simulink model "FBL_UAV_Final_All"  (R2024b)
settings: Solver=ode45  StartTime=0.0  StopTime=3  MaxStep=0.001  RelTol=1e-3
undefined symbols (not defined in the file): A, A_inv, B, Q, R
libraries: slpidlib x8, mpclib x1, rllib x1, simulink x1
(part 2 of 2)

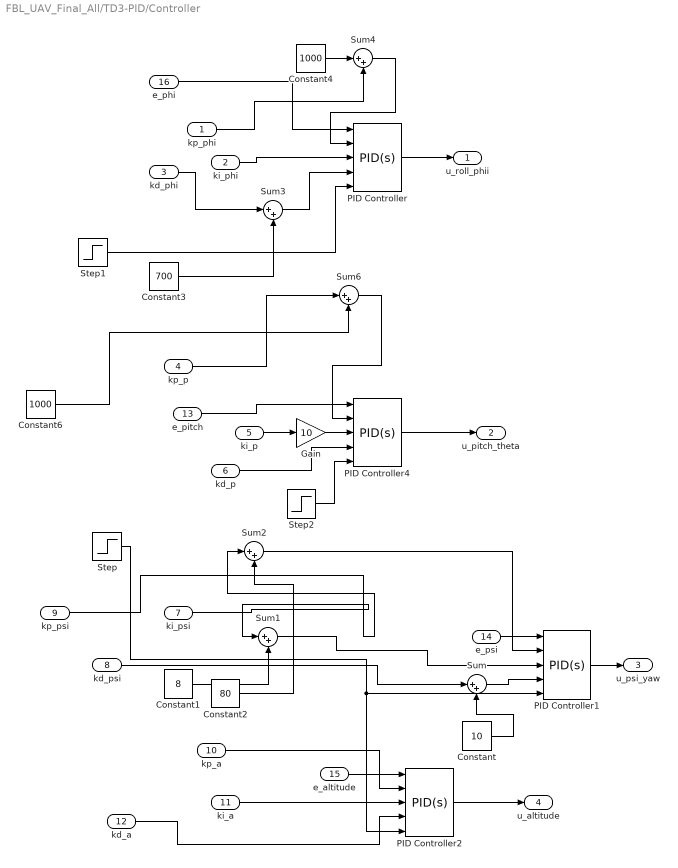
== system FBL_UAV_Final_All/TD3-PID/Controller ==
  kp_phi : Inport
  ki_phi : Inport  Port=2
  kd_phi : Inport  Port=3
  kp_p : Inport  Port=4
  ki_p : Inport  Port=5
  kd_p : Inport  Port=6
  ki_psi : Inport  Port=7
  kd_psi : Inport  Port=8
  kp_psi : Inport  Port=9
  kp_a : Inport  Port=10
  ki_a : Inport  Port=11
  kd_a : Inport  Port=12
  e_pitch : Inport  Port=13
  e_psi : Inport  Port=14
  e_altitude : Inport  Port=15
  e_phi : Inport  Port=16
  Constant : Constant  Value=10
  Constant1 : Constant  Value=8
  Constant2 : Constant  Value=80
  Constant3 : Constant  Value=700
  Constant4 : Constant  Value=1000
  Constant6 : Constant  Value=1000
  Gain : Gain  Gain=10
  PID Controller{,1..2,4} (4 alike) : slpidlib/PID Controller  Controller=PID  Form=Parallel  TimeDomain=Continuous-time  UseExternalTs=off  SampleTime=0.1  IntegratorMethod=Forward Euler  FilterMethod=Forward Euler  ControllerParametersSource=external  P=1  I=1  UseKiTs=off  D=0  UseExternalDerivativeSource=off  N=100  UseFilter=on  TunerSelectOption=Transfer Function Based (PID Tuner App)  InitialConditionSource=internal  InitialConditionForIntegrator=0  InitialConditionForFilter=0  DifferentiatorICPrevScaledInput=0  ExternalReset=none  TrackingMode=off  Kt=1  LimitOutput=off  SatLimitsSource=internal  UpperSaturationLimit=inf  LowerSaturationLimit=-inf  LinearizeAsGain=on  AntiWindupMode=none  Kb=1  LimitIntegrator=off  UpperIntegratorSaturationLimit=inf  LowerIntegratorSaturationLimit=-inf  POutMin=[]  POutMax=[]  IOutMin=[]  IOutMax=[]  DOutMin=[]  DOutMax=[]  NOutMin=[]  NOutMax=[]  SumOutMin=[]  SumOutMax=[]  SaturationOutMin=[]  SaturationOutMax=[]  PParamMin=[]  PParamMax=[]  IParamMin=[]  IParamMax=[]  DParamMin=[]  DParamMax=[]  NParamMin=[]  NParamMax=[]  KbParamMin=[]  KbParamMax=[]  KtParamMin=[]  KtParamMax=[]  KbOutMin=[]  KbOutMax=[]  KtOutMin=[]  KtOutMax=[]  IntegratorOutMin=[]  IntegratorOutMax=[]  FilterOutMin=[]  FilterOutMax=[]  SumI1OutMin=[]  SumI1OutMax=[]  SumI2OutMin=[]  SumI2OutMax=[]  SumI3OutMin=[]  SumI3OutMax=[]  SumI4OutMin=[]  SumI4OutMax=[]  SumDOutMin=[]  SumDOutMax=[]  DifferentiatorOutMin=[]  DifferentiatorOutMax=[]  FilterDiffOutCoefMin=[]  FilterDiffOutCoefMax=[]  ReciprocalOutMin=[]  ReciprocalOutMax=[]  SumDenOutMin=[]  SumDenOutMax=[]  SumNumOutMin=[]  SumNumOutMax=[]  DivideOutMin=[]  DivideOutMax=[]  UdiffTsProdOutMin=[]  UdiffTsProdOutMax=[]  NTsProdOutMin=[]  NTsProdOutMax=[]  UintegralTsProdOutMin=[]  UintegralTsProdOutMax=[]  UngainTsProdOutMin=[]  UngainTsProdOutMax=[]  ClampingZeroOutDataTypeStr=Inherit: Inherit via back propagation  ClampingZeroOutMin=[]  ClampingZeroOutMax=[]  FilterDenConstantOutDataTypeStr=Inherit: Inherit via back propagation  FilterDenConstantOutMin=[]  FilterDenConstantOutMax=[]  PCopyOutDataTypeStr=Inherit: Inherit via back propagation  PCopyOutMin=[]  PCopyOutMax=[]  NCopyOutDataTypeStr=Inherit: Inherit via back propagation  NCopyOutMin=[]  NCopyOutMax=[]  IntegratorContinuousStateAttributes=''  IntegratorStateMustResolveToSignalObject=off  IntegratorRTWStateStorageClass=Auto  FilterContinuousStateAttributes=''  FilterStateMustResolveToSignalObject=off  FilterRTWStateStorageClass=Auto  ParallelPVariant=ExternalParameters  IdealPVariant=Disabled  IVariant=ExternalParameters  DVariant=ExternalParameters  IntegratorVariant=Continuous  SatVariant=Disabled  AWVariant=Passthrough  PCopyVariant=Disabled  TRVariant=Disabled  FdbkBlocksVariant=Forward  IdealPFdbkVariant=Disabled  SatFdbkVariant=Disabled  DerivativeFilterVariant=ContFilter  NVariant=ExternalParameters  NCopyVariant=Disabled  FilterICVariant=InternalICsFilter  IntegratorICVariant=InternalICs  ExternalResetVariant=Disabled  TRSumVariant=Passthrough  SumFdbkVariant=Disabled  SumVariant=Sum_PID  TsampFilterVariant=InternalTs  TsampNgainVariant=Passthrough  TsampIntegralVariant=Disabled_SignalSpec  ExternalSaturationOutDataTypeStr=Inherit: Same as second input  DerivativeSourceVariant=ErrorSignal  PreIntVariant=InternalPreInt
  Step : Step  Time=0  After=800  SampleTime=0.1
  Step1 : Step  Time=0  After=800  SampleTime=0.1
  Step2 : Step  Time=0  After=700  SampleTime=0.1
  Sum{,1..4,6} (6 alike) : Sum  Inputs=|++
  u_roll_phii : Outport
  u_pitch_theta : Outport  Port=2
  u_psi_yaw : Outport  Port=3
  u_altitude : Outport  Port=4
  wires:
  Step/1 -> PID Controller2/5, PID Controller1/5
  e_phi/1 -> PID Controller/1
  PID Controller/1 -> u_roll_phii/1
  PID Controller4/1 -> u_pitch_theta/1
  PID Controller2/1 -> u_altitude/1
  e_altitude/1 -> PID Controller2/1
  e_psi/1 -> PID Controller1/1
  PID Controller1/1 -> u_psi_yaw/1
  kp_a/1 -> PID Controller2/2
  ki_a/1 -> PID Controller2/3
  kd_a/1 -> PID Controller2/4
  kp_psi/1 -> Sum2/1
  ki_psi/1 -> Sum1/1
  kd_psi/1 -> Sum/1
  Constant/1 -> Sum/2
  Sum/1 -> PID Controller1/4
  Constant1/1 -> Sum1/2
  Sum1/1 -> PID Controller1/3
  Sum2/1 -> PID Controller1/2
  Constant2/1 -> Sum2/2
  kp_phi/1 -> Sum4/2
  kd_phi/1 -> Sum3/1
  e_pitch/1 -> PID Controller4/1
  ki_p/1 -> Gain/1
  Step1/1 -> PID Controller/5
  Step2/1 -> PID Controller4/5
  kp_p/1 -> Sum6/1
  kd_p/1 -> PID Controller4/4
  Gain/1 -> PID Controller4/3
  Sum3/1 -> PID Controller/4
  Constant4/1 -> Sum4/1
  Sum4/1 -> PID Controller/2
  ki_phi/1 -> PID Controller/3
  Constant6/1 -> Sum6/2
  Sum6/1 -> PID Controller4/2
  Constant3/1 -> Sum3/2

== system FBL_UAV_Final_All/TD3-PID/IAE Calculation1 ==
  In1 : Inport
  Abs : Abs  SaturateOnIntegerOverflow=off
  Integrator6 : Integrator
  Out1 : Outport
  wires:
  Abs/1 -> Integrator6/1
  Integrator6/1 -> Out1/1
  In1/1 -> Abs/1

== system FBL_UAV_Final_All/TD3-PID/ISE Calculation_pitch ==
  In1 : Inport
  Integrator6 : Integrator
  Square : Math  Operator=square
  ISE : Outport
  wires:
  Square/1 -> Integrator6/1
  Integrator6/1 -> ISE/1
  In1/1 -> Square/1

== system FBL_UAV_Final_All/TD3-PID/ISE Calculation_roll ==
  In1 : Inport
  Integrator6 : Integrator
  Square : Math  Operator=square
  ISE : Outport
  wires:
  Square/1 -> Integrator6/1
  Integrator6/1 -> ISE/1
  In1/1 -> Square/1

== system FBL_UAV_Final_All/TD3-PID/ISE Calculation_yaw ==
  In1 : Inport
  Integrator6 : Integrator
  Square : Math  Operator=square
  ISE : Outport
  wires:
  Square/1 -> Integrator6/1
  Integrator6/1 -> ISE/1
  In1/1 -> Square/1

== system FBL_UAV_Final_All/TD3-PID/ISE Calculation_z ==
  In1 : Inport
  Integrator6 : Integrator
  Square : Math  Operator=square
  ISE : Outport
  wires:
  Square/1 -> Integrator6/1
  Integrator6/1 -> ISE/1
  In1/1 -> Square/1

== system FBL_UAV_Final_All/TD3-PID/RMSE Calculation_altitude ==
  In1 : Inport
  Gain : Gain  Gain=1/3435
  Memory : Memory
  Sqrt : Sqrt
  Square : Math  Operator=square
  Sum : Sum  Inputs=|++
  Out1 : Outport
  wires:
  In1/1 -> Square/1
  Square/1 -> Sum/1
  Memory/1 -> Sum/2
  Sum/1 -> Gain/1
  Gain/1 -> Sqrt/1, Memory/1
  Sqrt/1 -> Out1/1

== system FBL_UAV_Final_All/TD3-PID/RMSE Calculation_altitude1 ==
  In1 : Inport
  Gain : Gain  Gain=1/3435
  Memory : Memory
  Sqrt : Sqrt
  Square : Math  Operator=square
  Sum : Sum  Inputs=|++
  Out1 : Outport
  wires:
  In1/1 -> Square/1
  Square/1 -> Sum/1
  Memory/1 -> Sum/2
  Sum/1 -> Gain/1
  Gain/1 -> Sqrt/1, Memory/1
  Sqrt/1 -> Out1/1

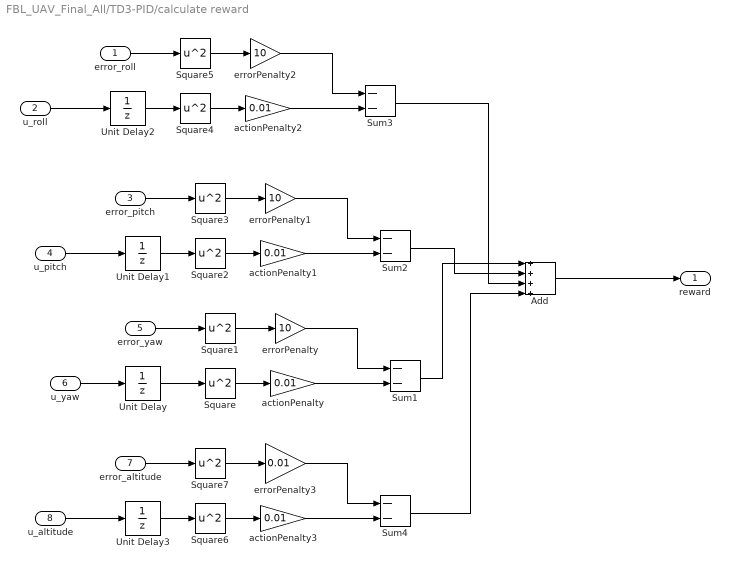
== system FBL_UAV_Final_All/TD3-PID/calculate reward ==
  error_roll : Inport
  u_roll : Inport  Port=2
  error_pitch : Inport  Port=3
  u_pitch : Inport  Port=4
  error_yaw : Inport  Port=5
  u_yaw : Inport  Port=6
  error_altitude : Inport  Port=7
  u_altitude : Inport  Port=8
  Add : Sum  Inputs=++++
  Square{,1..7} (8 alike) : Math  Operator=square
  Sum{1..4} (4 alike) : Sum  Inputs=--  OutDataTypeStr=double
  Unit Delay{,1..3} (4 alike) : UnitDelay  SampleTime=-1  HasFrameUpgradeWarning=on
  actionPenalty{,1..3} (4 alike) : Gain  Gain=0.01
  errorPenalty : Gain  Gain=10
  errorPenalty1 : Gain  Gain=10
  errorPenalty2 : Gain  Gain=10
  errorPenalty3 : Gain  Gain=0.01
  reward : Outport
  wires:
  Square1/1 -> errorPenalty/1
  errorPenalty/1 -> Sum1/1
  actionPenalty/1 -> Sum1/2
  Square/1 -> actionPenalty/1
  u_yaw/1 -> Unit Delay/1
  error_yaw/1 -> Square1/1
  Sum1/1 -> Add/1
  Square3/1 -> errorPenalty1/1
  Square2/1 -> actionPenalty1/1
  error_pitch/1 -> Square3/1
  u_pitch/1 -> Unit Delay1/1
  errorPenalty1/1 -> Sum2/1
  Sum2/1 -> Add/2
  actionPenalty1/1 -> Sum2/2
  Square5/1 -> errorPenalty2/1
  Square4/1 -> actionPenalty2/1
  error_roll/1 -> Square5/1
  u_roll/1 -> Unit Delay2/1
  errorPenalty2/1 -> Sum3/1
  Sum3/1 -> Add/3
  actionPenalty2/1 -> Sum3/2
  Square7/1 -> errorPenalty3/1
  Square6/1 -> actionPenalty3/1
  error_altitude/1 -> Square7/1
  u_altitude/1 -> Unit Delay3/1
  errorPenalty3/1 -> Sum4/1
  Sum4/1 -> Add/4
  actionPenalty3/1 -> Sum4/2
  Unit Delay/1 -> Square/1
  Unit Delay1/1 -> Square2/1
  Unit Delay2/1 -> Square4/1
  Unit Delay3/1 -> Square6/1
  Add/1 -> reward/1

== system FBL_UAV_Final_All/TD3-PID/error_altitude ==
  e : Inport
  Derivative : Derivative
  Integrator : Integrator
  p : Outport
  i : Outport  Port=2
  d : Outport  Port=3
  wires:
  Integrator/1 -> i/1
  e/1 -> Derivative/1, Integrator/1, p/1
  Derivative/1 -> d/1

== system FBL_UAV_Final_All/TD3-PID/error_phi_roll ==
  e : Inport
  Derivative : Derivative
  Integrator : Integrator
  p : Outport
  i : Outport  Port=2
  d : Outport  Port=3
  wires:
  Integrator/1 -> i/1
  e/1 -> p/1, Derivative/1, Integrator/1
  Derivative/1 -> d/1

== system FBL_UAV_Final_All/TD3-PID/error_pitch_theta ==
  e : Inport
  Derivative : Derivative
  Integrator : Integrator
  p : Outport
  i : Outport  Port=2
  d : Outport  Port=3
  wires:
  Integrator/1 -> i/1
  e/1 -> p/1, Derivative/1, Integrator/1
  Derivative/1 -> d/1

== system FBL_UAV_Final_All/TD3-PID/error_yaw_psi ==
  e : Inport
  Derivative : Derivative
  Integrator : Integrator
  p : Outport
  i : Outport  Port=2
  d : Outport  Port=3
  wires:
  Integrator/1 -> i/1
  e/1 -> p/1, Derivative/1, Integrator/1
  Derivative/1 -> d/1

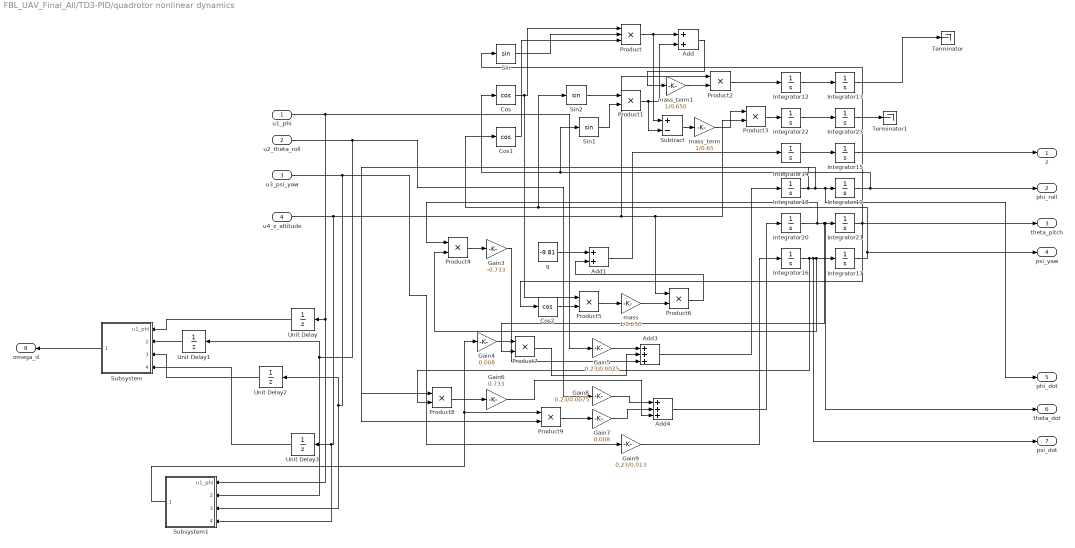
== system FBL_UAV_Final_All/TD3-PID/quadrotor nonlinear dynamics ==
  u1_phi : Inport
  u2_theta_roll : Inport  Port=2
  u3_psi_yaw : Inport  Port=3
  u4_z_altitude : Inport  Port=4
  Add : Sum
  Add1 : Sum
  Add3 : Sum  Inputs=+++
  Add4 : Sum  Inputs=+++
  Cos : Trigonometry  Operator=cos
  Cos1 : Trigonometry  Operator=cos
  Cos2 : Trigonometry  Operator=cos
  Gain3 : Gain  Gain=-0.733
  Gain4 : Gain  Gain=0.008
  Gain5 : Gain  Gain=0.23/0.0075
  Gain6 : Gain  Gain=0.733
  Gain7 : Gain  Gain=0.008
  Gain8 : Gain  Gain=0.23/0.0075
  Gain9 : Gain  Gain=0.23/0.013
  Integrator{12..15,18,20,22..23} (8 alike) : Integrator
  Integrator16 : Integrator  LowerSaturationLimit=0
  Integrator17 : Integrator  InitialCondition=1  LowerSaturationLimit=0
  Integrator19 : Integrator  InitialCondition=1  LowerSaturationLimit=0
  Integrator21 : Integrator  InitialCondition=1  LowerSaturationLimit=0
  Product : Product  Inputs=3
  Product{1..9} (9 alike) : Product
  Sin : Trigonometry
  Sin1 : Trigonometry
  Sin2 : Trigonometry
  Subsystem : Subsystem
  Subsystem1 : Subsystem
  Subtract : Sum  Inputs=+-
  Terminator : Terminator
  Terminator1 : Terminator
  Unit Delay{,1..3} (4 alike) : UnitDelay  SampleTime=-1  HasFrameUpgradeWarning=on
  g : Constant  Value=-9.81
  mass : Gain  Gain=1/0.650
  mass_term : Gain  Gain=1/0.65
  mass_term1 : Gain  Gain=1/0.650
  z : Outport
  phi_roll : Outport  Port=2
  theta_pitch : Outport  Port=3
  psi_yaw : Outport  Port=4
  phi_dot : Outport  Port=5
  theta_dot : Outport  Port=6
  psi_dot : Outport  Port=7
  omega_d : Outport  Port=8
  wires:
  Gain9/1 -> Integrator16/1
  Product9/1 -> Gain7/1
  Gain6/1 -> Add4/3
  Add3/1 -> Integrator18/1
  Add4/1 -> Integrator20/1
  Gain7/1 -> Add4/2
  Gain4/1 -> Product7/1
  Product7/1 -> Add3/2
  Product1/1 -> Subtract/2, Add/2
  g/1 -> Add1/1
  mass_term/1 -> Product3/1
  Integrator18/1 -> Product9/2, Product8/1, phi_dot/1, Integrator19/1
  mass/1 -> Product6/2
  Gain8/1 -> Add4/1
  mass_term1/1 -> Product2/2
  Gain5/1 -> Add3/1
  Product5/1 -> mass/1
  Integrator12/1 -> Integrator13/1
  Product/1 -> Subtract/1, Add/1
  Product2/1 -> Integrator12/1
  Integrator15/1 -> z/1
  Integrator22/1 -> Integrator23/1
  Add1/1 -> Integrator14/1
  Integrator14/1 -> Integrator15/1
  Cos1/1 -> Product/3
  Cos/1 -> Product5/1, Product/1
  Integrator17/1 -> Sin2/1, Cos1/1, psi_yaw/1
  Sin1/1 -> Product1/2
  Integrator20/1 -> theta_dot/1, Integrator21/1, Product7/2, Product4/1
  Integrator16/1 -> Product8/2, Product4/2, Integrator17/1, psi_dot/1
  Integrator21/1 -> theta_pitch/1, Cos2/1, Sin/1
  Add/1 -> mass_term1/1
  Product4/1 -> Gain3/1
  Product6/1 -> Add1/2
  Sin2/1 -> Product1/1
  Product8/1 -> Gain6/1
  Sin/1 -> Product/2
  Cos2/1 -> Product5/2
  Product3/1 -> Integrator22/1
  Subtract/1 -> mass_term/1
  Gain3/1 -> Add3/3
  Integrator19/1 -> Sin1/1, Cos/1, phi_roll/1
  u1_phi/1 -> Subsystem1/1(u1_phi), Unit Delay/1, Gain5/1
  u4_z_altitude/1 -> Product3/2, Product6/1, Product2/1, Subsystem1/4(u4_z_altitude), Unit Delay3/1
  u3_psi_yaw/1 -> Subsystem1/3(u3_psi_yaw), Unit Delay2/1, Gain9/1
  u2_theta_roll/1 -> Subsystem1/2(u2_theta_roll), Unit Delay1/1, Gain8/1
  Unit Delay/1 -> Subsystem/1(u1_phi)
  Unit Delay1/1 -> Subsystem/2(u2_theta_roll)
  Unit Delay2/1 -> Subsystem/3(u3_psi_yaw)
  Unit Delay3/1 -> Subsystem/4(u4_z_altitude)
  Integrator13/1 -> Terminator/1
  Integrator23/1 -> Terminator1/1
  Subsystem/1(omega_d) -> omega_d/1
  Subsystem1/1(omega_d) -> Product9/1, Gain4/1

== system FBL_UAV_Final_All/TD3-PID/square wave ==
  Scope : Scope
  Step : Step  Time=4  SampleTime=0
  Step1 : Step  Time=8  After=-1  SampleTime=0
  Step2 : Step  Time=10  After=-1  SampleTime=0
  Sum6 : Sum  Inputs=|++++
  new : Step  Time=2  SampleTime=0.1
  Out1 : Outport
  wires:
  Sum6/1 -> Out1/1, Scope/1
  Step/1 -> Sum6/2
  new/1 -> Sum6/1
  Step1/1 -> Sum6/3
  Step2/1 -> Sum6/4

== system FBL_UAV_Final_All/LMPC/quadrotor nonlinear dynamics/Subsystem ==
  u1_phi : Inport
  u2_theta_roll : Inport  Port=2
  u3_psi_yaw : Inport  Port=3
  u4_z_altitude : Inport  Port=4
  Constant2 : Constant  Value=A_inv
  Demux : Demux
  Matrix Multiply : Product  Multiplication=Matrix(*)
  Mux1 : Mux
  Saturation{,1..3} (4 alike) : Saturate  UpperLimit=490000  LowerLimit=0
  Sqrt{,1..3} (4 alike) : Sqrt
  Sum of Elements : Sum  Inputs=-+-+
  omega_d : Outport
  wires:
  Mux1/1 -> Matrix Multiply/2
  Saturation2/1 -> Sqrt2/1
  Demux/4 -> Saturation3/1
  u1_phi/1 -> Mux1/1
  Sqrt1/1 -> Sum of Elements/2
  Sqrt/1 -> Sum of Elements/1
  Saturation1/1 -> Sqrt1/1
  Constant2/1 -> Matrix Multiply/1
  Saturation/1 -> Sqrt/1
  Matrix Multiply/1 -> Demux/1
  Saturation3/1 -> Sqrt3/1
  Demux/2 -> Saturation1/1
  Demux/1 -> Saturation/1
  Demux/3 -> Saturation2/1
  Sqrt2/1 -> Sum of Elements/3
  u3_psi_yaw/1 -> Mux1/3
  u2_theta_roll/1 -> Mux1/2
  Sqrt3/1 -> Sum of Elements/4
  u4_z_altitude/1 -> Mux1/4
  Sum of Elements/1 -> omega_d/1

== system FBL_UAV_Final_All/LMPC/quadrotor nonlinear dynamics/Subsystem1 ==
  u1_phi : Inport
  u2_theta_roll : Inport  Port=2
  u3_psi_yaw : Inport  Port=3
  u4_z_altitude : Inport  Port=4
  Constant2 : Constant  Value=A_inv
  Demux : Demux
  Matrix Multiply : Product  Multiplication=Matrix(*)
  Mux1 : Mux
  Saturation{,1..3} (4 alike) : Saturate  UpperLimit=490000  LowerLimit=0
  Sqrt{,1..3} (4 alike) : Sqrt
  Sum of Elements : Sum  Inputs=-+-+
  omega_d : Outport
  wires:
  Mux1/1 -> Matrix Multiply/2
  Saturation2/1 -> Sqrt2/1
  Demux/4 -> Saturation3/1
  u1_phi/1 -> Mux1/1
  Sqrt1/1 -> Sum of Elements/2
  Sqrt/1 -> Sum of Elements/1
  Saturation1/1 -> Sqrt1/1
  Constant2/1 -> Matrix Multiply/1
  Saturation/1 -> Sqrt/1
  Matrix Multiply/1 -> Demux/1
  Saturation3/1 -> Sqrt3/1
  Demux/2 -> Saturation1/1
  Demux/1 -> Saturation/1
  Demux/3 -> Saturation2/1
  Sqrt2/1 -> Sum of Elements/3
  u3_psi_yaw/1 -> Mux1/3
  u2_theta_roll/1 -> Mux1/2
  Sqrt3/1 -> Sum of Elements/4
  u4_z_altitude/1 -> Mux1/4
  Sum of Elements/1 -> omega_d/1

== system FBL_UAV_Final_All/LQR/quadrotor nonlinear dynamics/Subsystem ==
  u1_phi : Inport
  u2_theta_roll : Inport  Port=2
  u3_psi_yaw : Inport  Port=3
  u4_z_altitude : Inport  Port=4
  Constant2 : Constant  Value=A_inv
  Demux : Demux
  Matrix Multiply : Product  Multiplication=Matrix(*)
  Mux1 : Mux
  Saturation{,1..3} (4 alike) : Saturate  UpperLimit=490000  LowerLimit=0
  Sqrt{,1..3} (4 alike) : Sqrt
  Sum of Elements : Sum  Inputs=-+-+
  omega_d : Outport
  wires:
  Mux1/1 -> Matrix Multiply/2
  Saturation2/1 -> Sqrt2/1
  Demux/4 -> Saturation3/1
  u1_phi/1 -> Mux1/1
  Sqrt1/1 -> Sum of Elements/2
  Sqrt/1 -> Sum of Elements/1
  Saturation1/1 -> Sqrt1/1
  Constant2/1 -> Matrix Multiply/1
  Saturation/1 -> Sqrt/1
  Matrix Multiply/1 -> Demux/1
  Saturation3/1 -> Sqrt3/1
  Demux/2 -> Saturation1/1
  Demux/1 -> Saturation/1
  Demux/3 -> Saturation2/1
  Sqrt2/1 -> Sum of Elements/3
  u3_psi_yaw/1 -> Mux1/3
  u2_theta_roll/1 -> Mux1/2
  Sqrt3/1 -> Sum of Elements/4
  u4_z_altitude/1 -> Mux1/4
  Sum of Elements/1 -> omega_d/1

== system FBL_UAV_Final_All/LQR/quadrotor nonlinear dynamics/Subsystem1 ==
  u1_phi : Inport
  u2_theta_roll : Inport  Port=2
  u3_psi_yaw : Inport  Port=3
  u4_z_altitude : Inport  Port=4
  Constant2 : Constant  Value=A_inv
  Demux : Demux
  Matrix Multiply : Product  Multiplication=Matrix(*)
  Mux1 : Mux
  Saturation{,1..3} (4 alike) : Saturate  UpperLimit=490000  LowerLimit=0
  Sqrt{,1..3} (4 alike) : Sqrt
  Sum of Elements : Sum  Inputs=-+-+
  omega_d : Outport
  wires:
  Mux1/1 -> Matrix Multiply/2
  Saturation2/1 -> Sqrt2/1
  Demux/4 -> Saturation3/1
  u1_phi/1 -> Mux1/1
  Sqrt1/1 -> Sum of Elements/2
  Sqrt/1 -> Sum of Elements/1
  Saturation1/1 -> Sqrt1/1
  Constant2/1 -> Matrix Multiply/1
  Saturation/1 -> Sqrt/1
  Matrix Multiply/1 -> Demux/1
  Saturation3/1 -> Sqrt3/1
  Demux/2 -> Saturation1/1
  Demux/1 -> Saturation/1
  Demux/3 -> Saturation2/1
  Sqrt2/1 -> Sum of Elements/3
  u3_psi_yaw/1 -> Mux1/3
  u2_theta_roll/1 -> Mux1/2
  Sqrt3/1 -> Sum of Elements/4
  u4_z_altitude/1 -> Mux1/4
  Sum of Elements/1 -> omega_d/1

== system FBL_UAV_Final_All/TD3-PID/quadrotor nonlinear dynamics/Subsystem ==
  u1_phi : Inport
  u2_theta_roll : Inport  Port=2
  u3_psi_yaw : Inport  Port=3
  u4_z_altitude : Inport  Port=4
  Constant2 : Constant  Value=A_inv
  Demux : Demux
  Matrix Multiply : Product  Multiplication=Matrix(*)
  Mux1 : Mux
  Saturation{,1..3} (4 alike) : Saturate  UpperLimit=490000  LowerLimit=0
  Sqrt{,1..3} (4 alike) : Sqrt
  Sum of Elements : Sum  Inputs=-+-+
  omega_d : Outport
  wires:
  Mux1/1 -> Matrix Multiply/2
  Saturation2/1 -> Sqrt2/1
  Demux/4 -> Saturation3/1
  u1_phi/1 -> Mux1/1
  Sqrt1/1 -> Sum of Elements/2
  Sqrt/1 -> Sum of Elements/1
  Saturation1/1 -> Sqrt1/1
  Constant2/1 -> Matrix Multiply/1
  Saturation/1 -> Sqrt/1
  Matrix Multiply/1 -> Demux/1
  Saturation3/1 -> Sqrt3/1
  Demux/2 -> Saturation1/1
  Demux/1 -> Saturation/1
  Demux/3 -> Saturation2/1
  Sqrt2/1 -> Sum of Elements/3
  u3_psi_yaw/1 -> Mux1/3
  u2_theta_roll/1 -> Mux1/2
  Sqrt3/1 -> Sum of Elements/4
  u4_z_altitude/1 -> Mux1/4
  Sum of Elements/1 -> omega_d/1

== system FBL_UAV_Final_All/TD3-PID/quadrotor nonlinear dynamics/Subsystem1 ==
  u1_phi : Inport
  u2_theta_roll : Inport  Port=2
  u3_psi_yaw : Inport  Port=3
  u4_z_altitude : Inport  Port=4
  Constant2 : Constant  Value=A_inv
  Demux : Demux
  Matrix Multiply : Product  Multiplication=Matrix(*)
  Mux1 : Mux
  Saturation{,1..3} (4 alike) : Saturate  UpperLimit=490000  LowerLimit=0
  Sqrt{,1..3} (4 alike) : Sqrt
  Sum of Elements : Sum  Inputs=-+-+
  omega_d : Outport
  wires:
  Mux1/1 -> Matrix Multiply/2
  Saturation2/1 -> Sqrt2/1
  Demux/4 -> Saturation3/1
  u1_phi/1 -> Mux1/1
  Sqrt1/1 -> Sum of Elements/2
  Sqrt/1 -> Sum of Elements/1
  Saturation1/1 -> Sqrt1/1
  Constant2/1 -> Matrix Multiply/1
  Saturation/1 -> Sqrt/1
  Matrix Multiply/1 -> Demux/1
  Saturation3/1 -> Sqrt3/1
  Demux/2 -> Saturation1/1
  Demux/1 -> Saturation/1
  Demux/3 -> Saturation2/1
  Sqrt2/1 -> Sum of Elements/3
  u3_psi_yaw/1 -> Mux1/3
  u2_theta_roll/1 -> Mux1/2
  Sqrt3/1 -> Sum of Elements/4
  u4_z_altitude/1 -> Mux1/4
  Sum of Elements/1 -> omega_d/1

== matlab function FBL_UAV_Final_All/LQR/inverse1 ==
  data: u input; y output
function y = fcn(u)

y = 1/u;

== matlab function FBL_UAV_Final_All/Fixed-Gain PID/inverse ==
  data: u input; y output
function y = fcn(u)

y = 1/u;

== matlab function FBL_UAV_Final_All/TD3-PID/MATLAB Function1 ==
  data: OutOfBounds input; cost output; ISE_z input; ISE_y input; ISE_p input; ISE_r input; t input; input_cost input
function cost = stoppingCriterion(OutOfBounds, ISE_z, ISE_y, ISE_p, ISE_r, t, input_cost)
simEndTime = 10;
epsilon = 0.05;

if OutOfBounds
    cost = input_cost-100;
elseif (t >= simEndTime - epsilon) && (ISE_z < 0.2) && (ISE_p < 0.2) && (ISE_y < 0.2) && (ISE_r < 0.2)
    cost = input_cost+10;
else
    cost = input_cost;
end

== matlab function FBL_UAV_Final_All/TD3-PID/inverse1 ==
  data: u input; y output
function y = fcn(u)

y = 1/u;

== matlab function FBL_UAV_Final_All/LMPC/inverse1 ==
  data: u input; y output
function y = fcn(u)

y = 1/u;
